simulink model "MDLL_sim"  (R2023b)
settings: Solver=VariableStepAuto  StartTime=0.0  StopTime=sim_time  RelTol=1e-3
values from neighbouring files (symbols this model uses):
  A0 = 5.7e-3    (= 0.0057)    [convmat_mdll.m]
  dco_white_free = 3e-5/10^1.4    (= 1.19432151166e-06)    [convmat_mdll.m]
  fdco = fref*N    (= 1600000000)    [convmat_mdll.m]
  fref = 50e6    (= 50000000)    [convmat_mdll.m]
  N = 32    [convmat_mdll.m]
  noise_dco_en = 1    [convmat_mdll.m]
  noise_ref_en = 1    [convmat_mdll.m]
  tdc_white_free = 3e-5/10^3.73    (= 5.58626140999e-09)    [convmat_mdll.m]
libraries: simulink x2
settings Model: Creator=frank  LastModifiedBy=koko35p
settings OptimizationCC: ReuseModelBlockBuffer=off

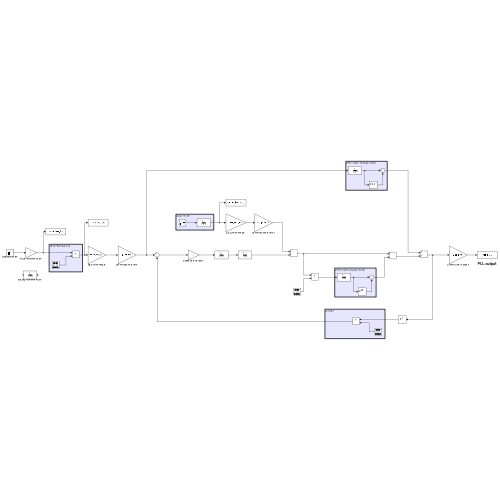
[thumbnail: Simulink's stored preview of the top-level diagram]
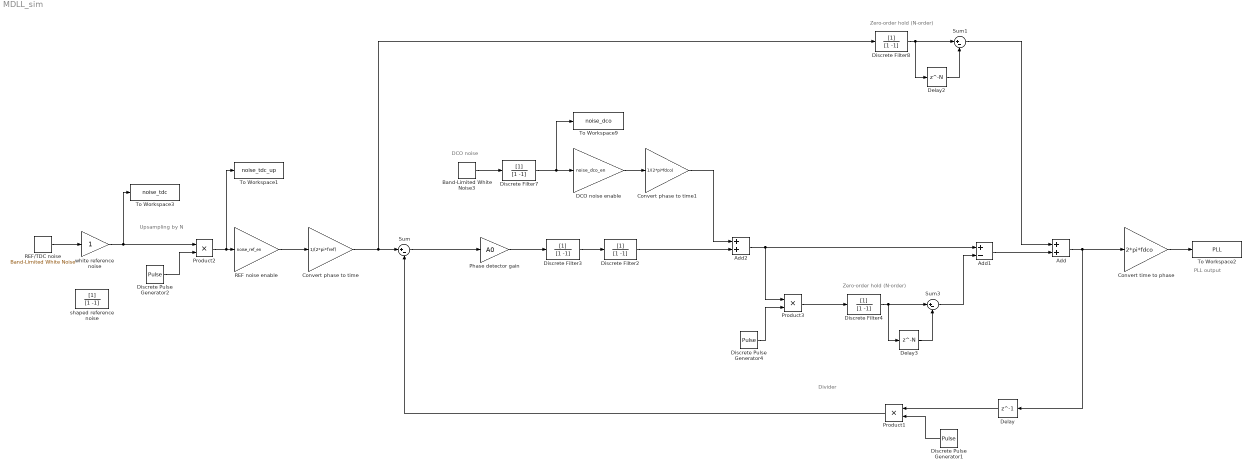
== system MDLL_sim ==
  note: DCO noise
  note: Divider
  note: Upsampling by N
  note: PLL output
  note: Zero-order hold (N-order)
  note: Zero-order hold (N-order)
  Add : Sum
  Add1 : Sum  Inputs=+-
  Add2 : Sum
  Band-Limited White Noise3 : simulink/Sources/Band-Limited White Noise  Cov=[dco_white_free/fdco]  Ts=1/fdco  seed=[446]
  Convert phase to time : Gain  Gain=1/(2*pi*fref)
  Convert phase to time1 : Gain  Gain=1/(2*pi*fdco)
  Convert time to phase : Gain  Gain=2*pi*fdco
  DCO noise enable : Gain  Gain=noise_dco_en
  Delay : Delay  DelayLength=1  InitialCondition=0
  Delay2 : Delay  DelayLength=N  InitialCondition=0
  Delay3 : Delay  DelayLength=N  InitialCondition=0
  Discrete Pulse Generator1 : DiscretePulseGenerator  Period=N  SampleTime=1/fdco
  Discrete Pulse Generator2 : DiscretePulseGenerator  Period=N  SampleTime=1/fdco
  Discrete Pulse Generator4 : DiscretePulseGenerator  Period=N  SampleTime=1/fdco
  Discrete Filter{2..4,7..8} (5 alike) : DiscreteFilter  Denominator=[1 -1]
  Phase detector gain : Gain  Gain=A0
  Product1 : Product
  Product2 : Product
  Product3 : Product
  REF noise enable : Gain  Gain=noise_ref_en
  REF/TDC noise : simulink/Sources/Band-Limited White Noise  Cov=[tdc_white_free/fref]  Ts=1/fref  seed=[486]
  Sum : Sum  Inputs=|+-
  Sum1 : Sum  Inputs=|+-
  Sum3 : Sum  Inputs=|+-
  To Workspace1 : ToWorkspace  VariableName=noise_tdc_up  SampleTime=-1
  To Workspace2 : ToWorkspace  VariableName=PLL  SampleTime=-1
  To Workspace3 : ToWorkspace  VariableName=noise_tdc  SampleTime=-1
  To Workspace9 : ToWorkspace  VariableName=noise_dco  SampleTime=-1
  shaped reference noise : DiscreteFilter  Denominator=[1 -1]
  white reference noise : Gain
  wires:
  Sum/1 -> Phase detector gain/1
  Add/1 -> Delay/1, Convert time to phase/1
  Discrete Pulse Generator1/1 -> Product1/2
  Discrete Pulse Generator2/1 -> Product2/2
  Band-Limited White Noise3/1 -> Discrete Filter7/1
  Discrete Filter7/1 -> To Workspace9/1, DCO noise enable/1
  Product1/1 -> Sum/2
  Discrete Filter3/1 -> Discrete Filter2/1
  Phase detector gain/1 -> Discrete Filter3/1
  Discrete Filter2/1 -> Add2/2
  Delay/1 -> Product1/1
  Sum1/1 -> Add/1
  Delay2/1 -> Sum1/2
  Discrete Filter8/1 -> Delay2/1, Sum1/1
  Add1/1 -> Add/2
  Add2/1 -> Add1/1, Product3/1
  Delay3/1 -> Sum3/2
  Discrete Filter4/1 -> Delay3/1, Sum3/1
  Discrete Pulse Generator4/1 -> Product3/2
  Product3/1 -> Discrete Filter4/1
  Sum3/1 -> Add1/2
  REF noise enable/1 -> Convert phase to time/1
  Convert phase to time/1 -> Discrete Filter8/1, Sum/1
  Convert time to phase/1 -> To Workspace2/1
  DCO noise enable/1 -> Convert phase to time1/1
  Convert phase to time1/1 -> Add2/1
  REF/TDC noise/1 -> white reference noise/1
  white reference noise/1 -> To Workspace3/1, Product2/1
  Product2/1 -> To Workspace1/1, REF noise enable/1
